simulink library "Enthalpy"  (Simulink 8.2)
settings: Solver=ode45  StartTime=0.0  StopTime=10.0  RelTol=1e-3
undefined symbols (not defined in the file): CarnotCallbacks_Enthalpy
settings Model: Creator=lena.frank  LastModifiedBy=drhf

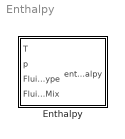
== system Enthalpy ==
  Enthalpy : Subsystem  LoadFcn=CarnotCallbacks_Enthalpy('LoadFcn');  InitFcn=load('THB.mat');  VariantControl=CarlibClassic  mask(enthalpy){INPUTARGUMENTS=state variables (classic), DEBUGLEVEL=WARNINGLEVEL, MAXTOTALMESSAGES=inf, MAXCONSECUTIVEMESSAGES=inf, WRITETOFILE=0, FILENAME='errors.txt'}
      mask prompts: INPUTARGUMENTS "Input arguments"; DEBUGLEVEL "Debug level"; MAXTOTALMESSAGES "maximum number of total warning"; MAXCONSECUTIVEMESSAGES "maximum number of consecutive warnings"; WRITETOFILE "write messages to file"; FILENAME "filename for error messages"
      mask help:
      | Calculates the fluid specific enthalpy  [J/kg].
      | Calls the CARNOT library "carlib".
      | WORKS FOR WATER AND DRY AIR! Enthalpy for other fluids is cp*T.
      | FluidType        Remarks
      | 1: water          fluid mix is vapourcontent in the 2-phase region
      | 2: air              fluid mix is (kg water) / (kg dry air)
      | 3: cotton oil       -
      | 4: silicone oil     -
      | 5: water-glycol   fluid mix is volume partition [0..1] of propylen glycol
      | 6: Tyfocor LS     function only available in liquid phase
      | 7: Water Constant = 0.0 J/kg (water at 20°C)
      | 8: Air Constant   = 0.0 J/kg (air at 20°C)
      mask init:
      | %Inports
      | CarnotCallbacks_Enthalpy('CreateInports');
      | 
      | %global debug level
      | [DEBUGLEVEL, MAXTOTALMESSAGES, MAXCONSECUTIVEMESSAGES, WRITETOFILE, FILENAME] = CarnotCallbacks_Enthalpy('CheckDebugLevels', DEBUGLEVEL, MAXTOTALMESSAGES, MAXCONSECUTIVEMESSAGES, WRITETOFILE, FILENAME);
      mask Help: web(fullfile(path_carnot('help'),'enthalpy.html'),'-helpbrowser')
      mask TypeOptions INPUTARGUMENTS: state variables (classic) | THB | THV
      mask Callback INPUTARGUMENTS: CarnotCallbacks_Enthalpy('MaskVisibilities');
      mask TypeOptions DEBUGLEVEL: DEBUGLEVEL | INFOLEVEL | WARNINGLEVEL | ERRORLEVEL | FATALLEVEL | NOLEVEL

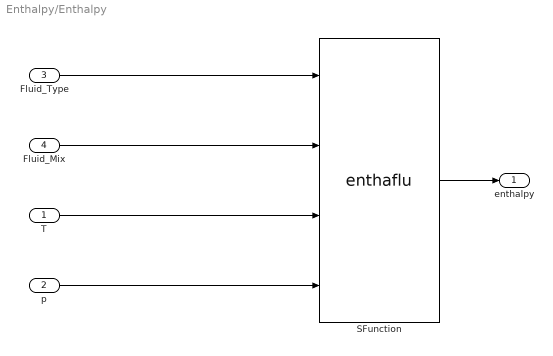
== system Enthalpy/Enthalpy ==
  T : Inport
  p : Inport  Port=2
  Fluid_Type : Inport  Port=3
  Fluid_Mix : Inport  Port=4
  SFunction : S-Function  FunctionName=enthaflu  Parameters=DEBUGLEVEL,MAXTOTALMESSAGES,MAXCONSECUTIVEMESSAGES,WRITETOFILE,FILENAME  EnableBusSupport=off
  enthalpy : Outport
  wires:
  SFunction/1 -> enthalpy/1
  T/1 -> SFunction/3
  p/1 -> SFunction/4
  Fluid_Type/1 -> SFunction/1
  Fluid_Mix/1 -> SFunction/2
